simulink model "Open_loop_BPS_comparsion2"  (R2023b)
settings: Solver=VariableStepAuto  StartTime=0.0  StopTime=10.0  RelTol=1e-3
undefined symbols (not defined in the file): X, Y, Z
libraries: nesl_utility x64, sm_lib x24
(part 1 of 2)
settings Model: Creator=msdbg  LastModifiedBy=msdbg

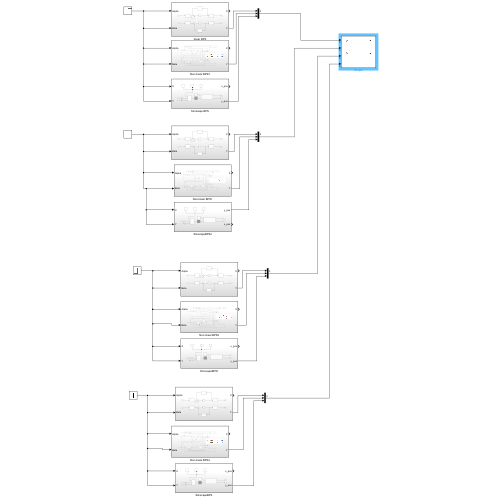
[thumbnail: Simulink's stored preview of the top-level diagram]
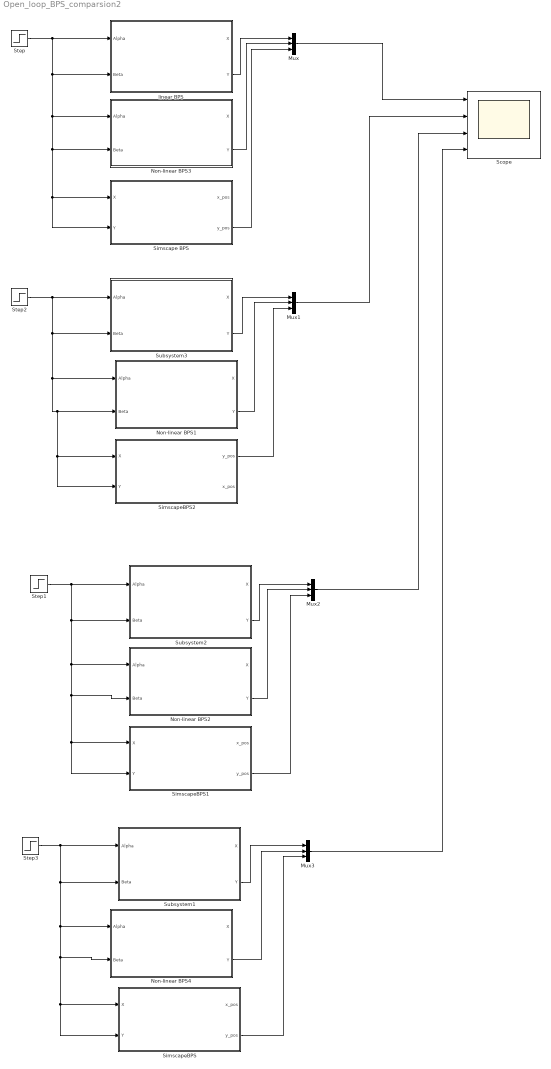
== system Open_loop_BPS_comparsion2 ==
  Mux{,1..3} (4 alike) : Mux  Inputs=3
  Non-linear BPS1 : Subsystem
  Non-linear BPS2 : Subsystem
  Non-linear BPS3 : Subsystem
  Non-linear BPS4 : Subsystem
  Scope : Scope  NumInputPorts=4
  Simscape BPS : Subsystem
  SimscapeBPS : Subsystem
  SimscapeBPS1 : Subsystem
  SimscapeBPS2 : Subsystem
  Step : Step  After=3.14/12  SampleTime=0
  Step1 : Step  After=3.14/8  SampleTime=0
  Step2 : Step  After=3.14/10  SampleTime=0
  Step3 : Step  After=3.14/6  SampleTime=0
  Subsystem1 : Subsystem
  Subsystem2 : Subsystem
  Subsystem3 : Subsystem
  linear BPS : Subsystem
  wires:
  Step3/1 -> Subsystem1/1(Alpha), Subsystem1/2(Beta), Non-linear BPS4/1(Alpha), Non-linear BPS4/2(Beta), SimscapeBPS/2(Y), SimscapeBPS/1(X)
  Mux3/1 -> Scope/4
  Mux/1 -> Scope/1
  Mux1/1 -> Scope/2
  Mux2/1 -> Scope/3
  Step1/1 -> Non-linear BPS2/1(Alpha), Non-linear BPS2/2(Beta), SimscapeBPS1/2(Y), SimscapeBPS1/1(X), Subsystem2/2(Beta), Subsystem2/1(Alpha)
  Step2/1 -> Non-linear BPS1/1(Alpha), Non-linear BPS1/2(Beta), SimscapeBPS2/2(Y), SimscapeBPS2/1(X), Subsystem3/2(Beta), Subsystem3/1(Alpha)
  Step/1 -> Simscape BPS/2(Y), Simscape BPS/1(X), Non-linear BPS3/2(Beta), Non-linear BPS3/1(Alpha), linear BPS/2(Beta), linear BPS/1(Alpha)
  Simscape BPS/2(y_pos) -> Mux/3
  Non-linear BPS1/2(Y) -> Mux1/2
  Non-linear BPS2/2(Y) -> Mux2/2
  Non-linear BPS4/2(Y) -> Mux3/2
  Non-linear BPS3/2(Y) -> Mux/2
  SimscapeBPS2/1(y_pos) -> Mux1/3
  SimscapeBPS1/2(y_pos) -> Mux2/3
  SimscapeBPS/2(y_pos) -> Mux3/3
  Subsystem1/2(Y) -> Mux3/1
  Subsystem2/2(Y) -> Mux2/1
  Subsystem3/2(Y) -> Mux1/1
  linear BPS/2(Y) -> Mux/1

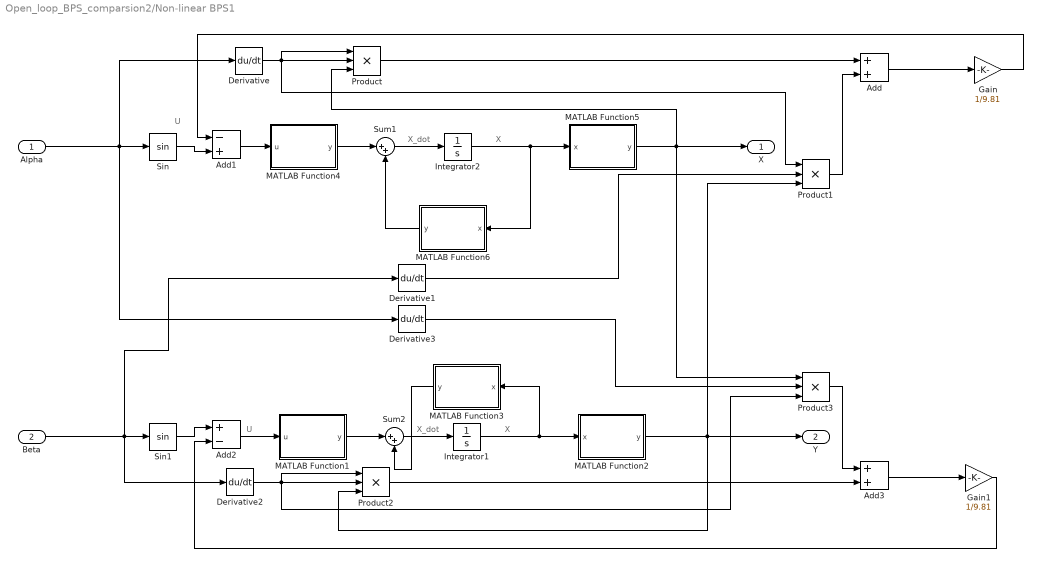
== system Open_loop_BPS_comparsion2/Non-linear BPS1 ==
  note: X
  note: U
  note: X_dot
  note: X_dot
  note: U
  note: X
  Alpha : Inport
  Beta : Inport  Port=2
  Add : Sum
  Add1 : Sum  Inputs=-+
  Add2 : Sum  Inputs=+-
  Add3 : Sum
  Derivative{,1..3} (4 alike) : Derivative
  Gain : Gain  Gain=1/9.81
  Gain1 : Gain  Gain=1/9.81
  Integrator1 : Integrator
  Integrator2 : Integrator
  MATLAB Function1 : MATLAB Function  TreatAsAtomicUnit=on
  MATLAB Function2 : MATLAB Function  TreatAsAtomicUnit=on
  MATLAB Function3 : MATLAB Function  TreatAsAtomicUnit=on
  MATLAB Function4 : MATLAB Function  TreatAsAtomicUnit=on
  MATLAB Function5 : MATLAB Function  TreatAsAtomicUnit=on
  MATLAB Function6 : MATLAB Function  TreatAsAtomicUnit=on
  Product{,1..3} (4 alike) : Product  Inputs=3
  Sin : Trigonometry
  Sin1 : Trigonometry
  Sum1 : Sum  Inputs=|++
  Sum2 : Sum  Inputs=|++
  X : Outport  PortDimensions=1
  Y : Outport  Port=2  PortDimensions=1
  wires:
  Beta/1 -> Sin1/1, Derivative1/1, Derivative2/1
  Alpha/1 -> Derivative3/1, Derivative/1, Sin/1
  Integrator2/1 -> MATLAB Function5/1(x), MATLAB Function6/1(x)
  MATLAB Function6/1(y) -> Sum1/2
  Integrator1/1 -> MATLAB Function2/1(x), MATLAB Function3/1(x)
  Product1/1 -> Add/2
  MATLAB Function3/1(y) -> Sum2/2
  MATLAB Function2/1(y) -> Y/1, Product1/3, Product2/3
  Gain1/1 -> Add2/2
  Derivative1/1 -> Product1/2
  MATLAB Function5/1(y) -> X/1, Product3/1, Product/3
  Add3/1 -> Gain1/1
  MATLAB Function4/1(y) -> Sum1/1
  Sin1/1 -> Add2/1
  Sum1/1 -> Integrator2/1
  MATLAB Function1/1(y) -> Sum2/1
  Derivative2/1 -> Product3/3, Product2/2, Product2/1
  Add/1 -> Gain/1
  Derivative/1 -> Product/1, Product1/1, Product/2
  Add2/1 -> MATLAB Function1/1(u)
  Sin/1 -> Add1/2
  Add1/1 -> MATLAB Function4/1(u)
  Derivative3/1 -> Product3/2
  Product2/1 -> Add3/2
  Sum2/1 -> Integrator1/1
  Product/1 -> Add/1
  Product3/1 -> Add3/1
  Gain/1 -> Add1/1

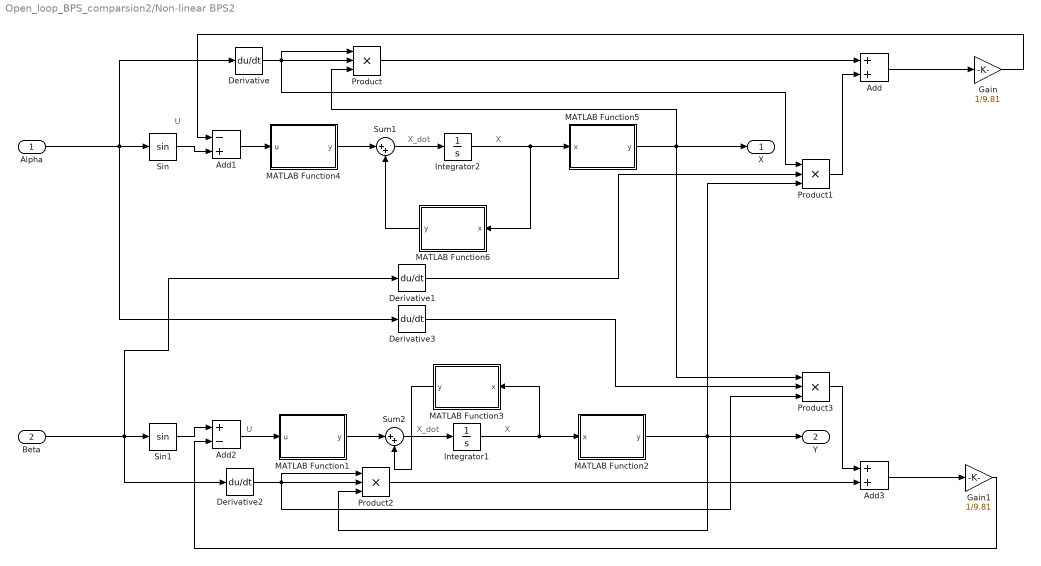
== system Open_loop_BPS_comparsion2/Non-linear BPS2 ==
  note: X
  note: U
  note: X_dot
  note: X_dot
  note: U
  note: X
  Alpha : Inport
  Beta : Inport  Port=2
  Add : Sum
  Add1 : Sum  Inputs=-+
  Add2 : Sum  Inputs=+-
  Add3 : Sum
  Derivative{,1..3} (4 alike) : Derivative
  Gain : Gain  Gain=1/9.81
  Gain1 : Gain  Gain=1/9.81
  Integrator1 : Integrator
  Integrator2 : Integrator
  MATLAB Function1 : MATLAB Function  TreatAsAtomicUnit=on
  MATLAB Function2 : MATLAB Function  TreatAsAtomicUnit=on
  MATLAB Function3 : MATLAB Function  TreatAsAtomicUnit=on
  MATLAB Function4 : MATLAB Function  TreatAsAtomicUnit=on
  MATLAB Function5 : MATLAB Function  TreatAsAtomicUnit=on
  MATLAB Function6 : MATLAB Function  TreatAsAtomicUnit=on
  Product{,1..3} (4 alike) : Product  Inputs=3
  Sin : Trigonometry
  Sin1 : Trigonometry
  Sum1 : Sum  Inputs=|++
  Sum2 : Sum  Inputs=|++
  X : Outport  PortDimensions=1
  Y : Outport  Port=2  PortDimensions=1
  wires:
  Beta/1 -> Sin1/1, Derivative1/1, Derivative2/1
  Alpha/1 -> Derivative3/1, Derivative/1, Sin/1
  Integrator2/1 -> MATLAB Function5/1(x), MATLAB Function6/1(x)
  MATLAB Function6/1(y) -> Sum1/2
  Integrator1/1 -> MATLAB Function2/1(x), MATLAB Function3/1(x)
  Product1/1 -> Add/2
  MATLAB Function3/1(y) -> Sum2/2
  MATLAB Function2/1(y) -> Y/1, Product1/3, Product2/3
  Gain1/1 -> Add2/2
  Derivative1/1 -> Product1/2
  MATLAB Function5/1(y) -> X/1, Product3/1, Product/3
  Add3/1 -> Gain1/1
  MATLAB Function4/1(y) -> Sum1/1
  Sin1/1 -> Add2/1
  Sum1/1 -> Integrator2/1
  MATLAB Function1/1(y) -> Sum2/1
  Derivative2/1 -> Product3/3, Product2/2, Product2/1
  Add/1 -> Gain/1
  Derivative/1 -> Product/1, Product1/1, Product/2
  Add2/1 -> MATLAB Function1/1(u)
  Sin/1 -> Add1/2
  Add1/1 -> MATLAB Function4/1(u)
  Derivative3/1 -> Product3/2
  Product2/1 -> Add3/2
  Sum2/1 -> Integrator1/1
  Product/1 -> Add/1
  Product3/1 -> Add3/1
  Gain/1 -> Add1/1

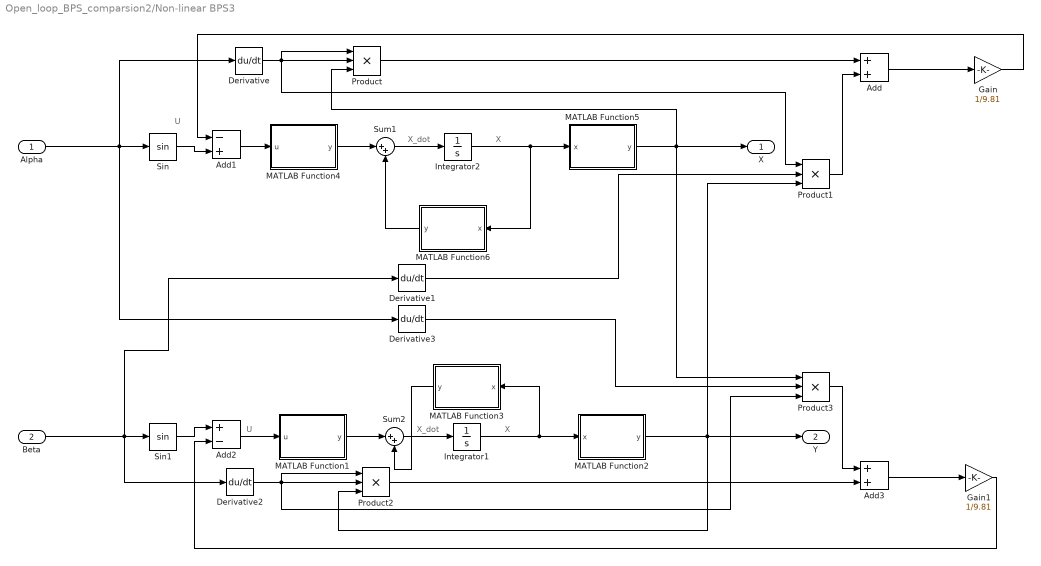
== system Open_loop_BPS_comparsion2/Non-linear BPS3 ==
  note: X
  note: U
  note: X_dot
  note: X_dot
  note: U
  note: X
  Alpha : Inport
  Beta : Inport  Port=2
  Add : Sum
  Add1 : Sum  Inputs=-+
  Add2 : Sum  Inputs=+-
  Add3 : Sum
  Derivative{,1..3} (4 alike) : Derivative
  Gain : Gain  Gain=1/9.81
  Gain1 : Gain  Gain=1/9.81
  Integrator1 : Integrator
  Integrator2 : Integrator
  MATLAB Function1 : MATLAB Function  TreatAsAtomicUnit=on
  MATLAB Function2 : MATLAB Function  TreatAsAtomicUnit=on
  MATLAB Function3 : MATLAB Function  TreatAsAtomicUnit=on
  MATLAB Function4 : MATLAB Function  TreatAsAtomicUnit=on
  MATLAB Function5 : MATLAB Function  TreatAsAtomicUnit=on
  MATLAB Function6 : MATLAB Function  TreatAsAtomicUnit=on
  Product{,1..3} (4 alike) : Product  Inputs=3
  Sin : Trigonometry
  Sin1 : Trigonometry
  Sum1 : Sum  Inputs=|++
  Sum2 : Sum  Inputs=|++
  X : Outport  PortDimensions=1
  Y : Outport  Port=2  PortDimensions=1
  wires:
  Beta/1 -> Sin1/1, Derivative1/1, Derivative2/1
  Alpha/1 -> Derivative3/1, Derivative/1, Sin/1
  Integrator2/1 -> MATLAB Function5/1(x), MATLAB Function6/1(x)
  MATLAB Function6/1(y) -> Sum1/2
  Integrator1/1 -> MATLAB Function2/1(x), MATLAB Function3/1(x)
  Product1/1 -> Add/2
  MATLAB Function3/1(y) -> Sum2/2
  MATLAB Function2/1(y) -> Y/1, Product1/3, Product2/3
  Gain1/1 -> Add2/2
  Derivative1/1 -> Product1/2
  MATLAB Function5/1(y) -> X/1, Product3/1, Product/3
  Add3/1 -> Gain1/1
  MATLAB Function4/1(y) -> Sum1/1
  Sin1/1 -> Add2/1
  Sum1/1 -> Integrator2/1
  MATLAB Function1/1(y) -> Sum2/1
  Derivative2/1 -> Product3/3, Product2/2, Product2/1
  Add/1 -> Gain/1
  Derivative/1 -> Product/1, Product1/1, Product/2
  Add2/1 -> MATLAB Function1/1(u)
  Sin/1 -> Add1/2
  Add1/1 -> MATLAB Function4/1(u)
  Derivative3/1 -> Product3/2
  Product2/1 -> Add3/2
  Sum2/1 -> Integrator1/1
  Product/1 -> Add/1
  Product3/1 -> Add3/1
  Gain/1 -> Add1/1

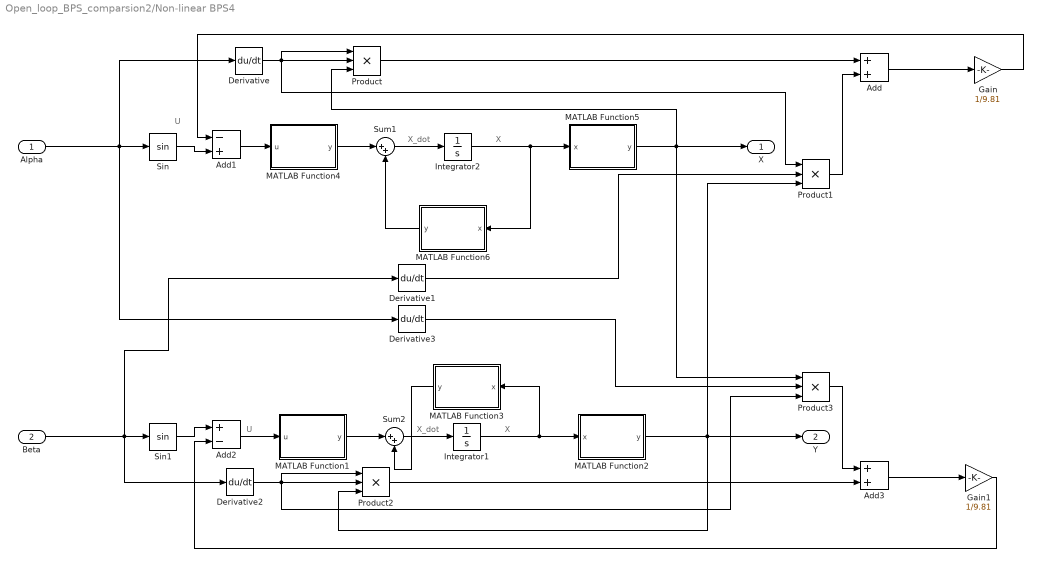
== system Open_loop_BPS_comparsion2/Non-linear BPS4 ==
  note: X
  note: U
  note: X_dot
  note: X_dot
  note: U
  note: X
  Alpha : Inport
  Beta : Inport  Port=2
  Add : Sum
  Add1 : Sum  Inputs=-+
  Add2 : Sum  Inputs=+-
  Add3 : Sum
  Derivative{,1..3} (4 alike) : Derivative
  Gain : Gain  Gain=1/9.81
  Gain1 : Gain  Gain=1/9.81
  Integrator1 : Integrator
  Integrator2 : Integrator
  MATLAB Function1 : MATLAB Function  TreatAsAtomicUnit=on
  MATLAB Function2 : MATLAB Function  TreatAsAtomicUnit=on
  MATLAB Function3 : MATLAB Function  TreatAsAtomicUnit=on
  MATLAB Function4 : MATLAB Function  TreatAsAtomicUnit=on
  MATLAB Function5 : MATLAB Function  TreatAsAtomicUnit=on
  MATLAB Function6 : MATLAB Function  TreatAsAtomicUnit=on
  Product{,1..3} (4 alike) : Product  Inputs=3
  Sin : Trigonometry
  Sin1 : Trigonometry
  Sum1 : Sum  Inputs=|++
  Sum2 : Sum  Inputs=|++
  X : Outport  PortDimensions=1
  Y : Outport  Port=2  PortDimensions=1
  wires:
  Beta/1 -> Sin1/1, Derivative1/1, Derivative2/1
  Alpha/1 -> Derivative3/1, Derivative/1, Sin/1
  Integrator2/1 -> MATLAB Function5/1(x), MATLAB Function6/1(x)
  MATLAB Function6/1(y) -> Sum1/2
  Integrator1/1 -> MATLAB Function2/1(x), MATLAB Function3/1(x)
  Product1/1 -> Add/2
  MATLAB Function3/1(y) -> Sum2/2
  MATLAB Function2/1(y) -> Y/1, Product1/3, Product2/3
  Gain1/1 -> Add2/2
  Derivative1/1 -> Product1/2
  MATLAB Function5/1(y) -> X/1, Product3/1, Product/3
  Add3/1 -> Gain1/1
  MATLAB Function4/1(y) -> Sum1/1
  Sin1/1 -> Add2/1
  Sum1/1 -> Integrator2/1
  MATLAB Function1/1(y) -> Sum2/1
  Derivative2/1 -> Product3/3, Product2/2, Product2/1
  Add/1 -> Gain/1
  Derivative/1 -> Product/1, Product1/1, Product/2
  Add2/1 -> MATLAB Function1/1(u)
  Sin/1 -> Add1/2
  Add1/1 -> MATLAB Function4/1(u)
  Derivative3/1 -> Product3/2
  Product2/1 -> Add3/2
  Sum2/1 -> Integrator1/1
  Product/1 -> Add/1
  Product3/1 -> Add3/1
  Gain/1 -> Add1/1

== system Open_loop_BPS_comparsion2/Simscape BPS ==
  X : Inport
  Y : Inport  Port=2
  Ball : sm_lib/Body Elements/Spherical Solid  GraphicAmbientColor=[0.15 0.15 0.15 1.0]  BasedOnType=Mass  CenterOfMass=[0 0 0]  CenterOfMassUnits=m  GraphicDiffuseColor=[0.5 0.5 0.5]  Density=1000  DensityUnits=kg/m^3  DoExposeReferenceFrame=on  GraphicEmissiveColor=[0.0 0.0 0.0 1.0]  ExportEntireGeometry=off  SerializedExposedGeometries=<exposedGeometries/>  SerializedFrames=<Frames/>  MarkerShape=Sphere  MarkerSize=10  GraphicType=FromGeometry  InertiaType=CalculateFromGeometry  Mass=51  MassUnits=g  MomentsOfInertia=[1 1 1]  MomentsOfInertiaUnits=kg*m^2  GraphicOpacity=1.0  ProductsOfInertia=[0 0 0]  ProductsOfInertiaUnits=kg*m^2  GraphicShininess=75  GraphicSpecularColor=[0.5 0.5 0.5 1.0]  SphereRadius=2.54/2  SphereRadiusUnits=cm  GraphicVisPropType=SimpleVisualProperties
  Ball Plate Interaction : Subsystem
  Mechanism Configuration : sm_lib/Utilities/Mechanism Configuration  UniformGravity=Constant  GravityVector=[0 0 -9.81]  GravityVectorUnits=m/s^2  LinearizationDelta=0.001  JointModeTransitionNonlinearIterations=2
  Plate : Subsystem
  Simulink-PS Converter : nesl_utility/Simulink-PS Converter  PhysicalDomain=network_engine_domain  SubClassName=ps_input  LeftPortType=input  RightPortType=output  PseudoPeriodic=off  Frequencies=[]  NoiseDistribution=none  NoiseParameters=[]  Unit=1  AffineConversion=off  FilteringAndDerivatives=zero  SimscapeFilterOrder=1  InputFilterTimeConstant=0.001  UdotUserProvided=0
  Simulink-PS Converter1 : nesl_utility/Simulink-PS Converter  PhysicalDomain=network_engine_domain  SubClassName=ps_input  LeftPortType=input  RightPortType=output  PseudoPeriodic=off  Frequencies=[]  NoiseDistribution=none  NoiseParameters=[]  Unit=1  AffineConversion=off  FilteringAndDerivatives=zero  SimscapeFilterOrder=1  InputFilterTimeConstant=0.001  UdotUserProvided=0
  Solver Configuration : nesl_utility/Solver Configuration  PhysicalDomain=network_engine_domain  SubClassName=solver  LeftPortType=input  RightPortType=generic  Tones=[]  Harmonics=[]  SimulateNoise=off  Profile=off  UseLocalSampling=off  EnableSwitchedLinearOptims=on  FrequencyDomain=off  UseCCode=off  RelTol=0.001  AbsTol=1e-06  MinStep=1e-09  ToWorkspace=off  RevertToSquareIcSolve=off  NumHomotopyIterations=100  PhasorMode=off  PhasorModeNumHarmonics=1  ConsistencySolver=NEWTON_FTOL  IndexReductionMethod=DerivativeReplacement  DoDC=off  ResidualTolerance=1e-9  ConsistencyTolSource=GLOBAL  ConsistencyAbsTol=0.001  ConsistencyRelTol=0.001  ConsistencyTolFactor=0.001  UseLocalSolver=off  LocalSolverChoice=NE_BACKWARD_EULER_ADVANCER  ResolveIndetEquations=on  FunctionEvalNumThread=1  LocalSolverSampleTime=.001  DoFixedCost=off  MaxNonlinIter=3  MaxModeIter=2  ComputeImpulses=off  ImpulseIterations=2  LinearAlgebra=Sparse  LinearAlgebraNumThread=0  EquationFormulation=NE_TIME_EF  DelaysMemoryBudget=1024  AutomaticFiltering=on  FilteringTimeConstant=0.001  PartitionStorageMethod=AS_NEEDED  PartitionMemoryBudget=1024  PartitionMethod=FAST  MultibodyUseLocalSolver=off  MultibodyLocalSolverChoice=ODE1  MultibodyLocalSolverSampleTime=0.001
  Universal Joint : sm_lib/Joints/Universal Joint  JointMode=Normal  SenseConstraintForce=off  SenseConstraintForceX=off  SenseConstraintForceY=off  SenseConstraintForceZ=off  SenseConstraintTorque=off  SenseConstraintTorqueX=off  SenseConstraintTorqueY=off  SenseConstraintTorqueZ=off  SenseTotalForce=off  SenseTotalForceX=off  SenseTotalForceY=off  SenseTotalForceZ=off  SenseTotalTorque=off  SenseTotalTorqueX=off  SenseTotalTorqueY=off  SenseTotalTorqueZ=off  CompositeWrenchDir=FollowerOnBase  CompositeWrenchFrame=BaseFrame  RxEquilibriumPosition=0  RxEquilibriumPositionUnits=deg  RxSpringStiffness=0  RxSpringStiffnessUnits=N*m/deg  RxDampingCoefficient=0  RxDampingCoefficientUnits=N*m/(deg/s)  RxTorqueActuationMode=ComputedTorque  RxMotionActuationMode=InputMotion  RxSensePosition=off  RxSenseVelocity=off  RxSenseAcceleration=off  RxSenseTorqueForce=off  RxSenseLowerLimitTorqueForce=off  RxSenseUpperLimitTorqueForce=off  RxLowerLimitSpecify=off  RxLowerLimitBound=-90  RxLowerLimitBoundUnits=deg  RxLowerLimitStiffness=1e4  RxLowerLimitStiffnessUnits=N*m/deg  RxLowerLimitDamping=10  RxLowerLimitDampingUnits=N*m/(deg/s)  RxLowerLimitTransitionRegionWidth=0.1  RxLowerLimitTransitionRegionWidthUnits=deg  RxUpperLimitSpecify=off  RxUpperLimitBound=90  RxUpperLimitBoundUnits=deg  RxUpperLimitStiffness=1e4  RxUpperLimitStiffnessUnits=N*m/deg  RxUpperLimitDamping=10  RxUpperLimitDampingUnits=N*m/(deg/s)  RxUpperLimitTransitionRegionWidth=0.1  RxUpperLimitTransitionRegionWidthUnits=deg  RxPositionTargetSpecify=off  RxPositionTargetPriority=High  RxPositionTargetValue=0  RxPositionTargetValueUnits=deg  RxVelocityTargetSpecify=off  RxVelocityTargetPriority=High  RxVelocityTargetValue=0  RxVelocityTargetValueUnits=deg/s  RyEquilibriumPosition=0  RyEquilibriumPositionUnits=deg  RySpringStiffness=0  RySpringStiffnessUnits=N*m/deg  RyDampingCoefficient=0  RyDampingCoefficientUnits=N*m/(deg/s)  RyTorqueActuationMode=ComputedTorque  RyMotionActuationMode=InputMotion  RySensePosition=off  RySenseVelocity=off  RySenseAcceleration=off  RySenseTorqueForce=off  RySenseLowerLimitTorqueForce=off  RySenseUpperLimitTorqueForce=off  RyLowerLimitSpecify=off  RyLowerLimitBound=-90  RyLowerLimitBoundUnits=deg  RyLowerLimitStiffness=1e4  RyLowerLimitStiffnessUnits=N*m/deg  RyLowerLimitDamping=10  RyLowerLimitDampingUnits=N*m/(deg/s)  RyLowerLimitTransitionRegionWidth=0.1  RyLowerLimitTransitionRegionWidthUnits=deg  RyUpperLimitSpecify=off  RyUpperLimitBound=90  RyUpperLimitBoundUnits=deg  RyUpperLimitStiffness=1e4  RyUpperLimitStiffnessUnits=N*m/deg  RyUpperLimitDamping=10  RyUpperLimitDampingUnits=N*m/(deg/s)  RyUpperLimitTransitionRegionWidth=0.1  RyUpperLimitTransitionRegionWidthUnits=deg  RyPositionTargetSpecify=off  RyPositionTargetPriority=High  RyPositionTargetValue=0  RyPositionTargetValueUnits=deg  RyVelocityTargetSpecify=off  RyVelocityTargetPriority=High  RyVelocityTargetValue=0  RyVelocityTargetValueUnits=deg/s
  World Frame : sm_lib/Frames and Transforms/World Frame
  x_pos : Outport  VectorParamsAs1DForOutWhenUnconnected=off
  y_pos : Outport  Port=2  VectorParamsAs1DForOutWhenUnconnected=off
  wires:
  Ball Plate Interaction/2(y_pos) -> y_pos/1
  X/1 -> Simulink-PS Converter/1
  Y/1 -> Simulink-PS Converter1/1
  Ball Plate Interaction/1(x_pos) -> x_pos/1
  connections:
  Plate/RConn1 -- Ball Plate Interaction/LConn2
  Mechanism Configuration/RConn1 -- Solver Configuration/RConn1 -- Universal Joint/LConn1 -- World Frame/RConn1
  Simulink-PS Converter/RConn1 -- Universal Joint/LConn2
  Plate/LConn1 -- Universal Joint/RConn1
  Simulink-PS Converter1/RConn1 -- Universal Joint/LConn3
  Ball Plate Interaction/LConn1 -- Ball/RConn1

== system Open_loop_BPS_comparsion2/SimscapeBPS ==
  X : Inport
  Y : Inport  Port=2
  Ball : sm_lib/Body Elements/Spherical Solid  GraphicAmbientColor=[0.15 0.15 0.15 1.0]  BasedOnType=Mass  CenterOfMass=[0 0 0]  CenterOfMassUnits=m  GraphicDiffuseColor=[0.5 0.5 0.5]  Density=1000  DensityUnits=kg/m^3  DoExposeReferenceFrame=on  GraphicEmissiveColor=[0.0 0.0 0.0 1.0]  ExportEntireGeometry=off  SerializedExposedGeometries=<exposedGeometries/>  SerializedFrames=<Frames/>  MarkerShape=Sphere  MarkerSize=10  GraphicType=FromGeometry  InertiaType=CalculateFromGeometry  Mass=51  MassUnits=g  MomentsOfInertia=[1 1 1]  MomentsOfInertiaUnits=kg*m^2  GraphicOpacity=1.0  ProductsOfInertia=[0 0 0]  ProductsOfInertiaUnits=kg*m^2  GraphicShininess=75  GraphicSpecularColor=[0.5 0.5 0.5 1.0]  SphereRadius=2.54/2  SphereRadiusUnits=cm  GraphicVisPropType=SimpleVisualProperties
  Ball Plate Interaction : Subsystem
  Mechanism Configuration : sm_lib/Utilities/Mechanism Configuration  UniformGravity=Constant  GravityVector=[0 0 -9.81]  GravityVectorUnits=m/s^2  LinearizationDelta=0.001  JointModeTransitionNonlinearIterations=2
  Plate : Subsystem
  Simulink-PS Converter : nesl_utility/Simulink-PS Converter  PhysicalDomain=network_engine_domain  SubClassName=ps_input  LeftPortType=input  RightPortType=output  PseudoPeriodic=off  Frequencies=[]  NoiseDistribution=none  NoiseParameters=[]  Unit=1  AffineConversion=off  FilteringAndDerivatives=zero  SimscapeFilterOrder=1  InputFilterTimeConstant=0.001  UdotUserProvided=0
  Simulink-PS Converter1 : nesl_utility/Simulink-PS Converter  PhysicalDomain=network_engine_domain  SubClassName=ps_input  LeftPortType=input  RightPortType=output  PseudoPeriodic=off  Frequencies=[]  NoiseDistribution=none  NoiseParameters=[]  Unit=1  AffineConversion=off  FilteringAndDerivatives=zero  SimscapeFilterOrder=1  InputFilterTimeConstant=0.001  UdotUserProvided=0
  Solver Configuration : nesl_utility/Solver Configuration  PhysicalDomain=network_engine_domain  SubClassName=solver  LeftPortType=input  RightPortType=generic  Tones=[]  Harmonics=[]  SimulateNoise=off  Profile=off  UseLocalSampling=off  EnableSwitchedLinearOptims=on  FrequencyDomain=off  UseCCode=off  RelTol=0.001  AbsTol=1e-06  MinStep=1e-09  ToWorkspace=off  RevertToSquareIcSolve=off  NumHomotopyIterations=100  PhasorMode=off  PhasorModeNumHarmonics=1  ConsistencySolver=NEWTON_FTOL  IndexReductionMethod=DerivativeReplacement  DoDC=off  ResidualTolerance=1e-9  ConsistencyTolSource=GLOBAL  ConsistencyAbsTol=0.001  ConsistencyRelTol=0.001  ConsistencyTolFactor=0.001  UseLocalSolver=off  LocalSolverChoice=NE_BACKWARD_EULER_ADVANCER  ResolveIndetEquations=on  FunctionEvalNumThread=1  LocalSolverSampleTime=.001  DoFixedCost=off  MaxNonlinIter=3  MaxModeIter=2  ComputeImpulses=off  ImpulseIterations=2  LinearAlgebra=Sparse  LinearAlgebraNumThread=0  EquationFormulation=NE_TIME_EF  DelaysMemoryBudget=1024  AutomaticFiltering=on  FilteringTimeConstant=0.001  PartitionStorageMethod=AS_NEEDED  PartitionMemoryBudget=1024  PartitionMethod=FAST  MultibodyUseLocalSolver=off  MultibodyLocalSolverChoice=ODE1  MultibodyLocalSolverSampleTime=0.001
  Universal Joint : sm_lib/Joints/Universal Joint  JointMode=Normal  SenseConstraintForce=off  SenseConstraintForceX=off  SenseConstraintForceY=off  SenseConstraintForceZ=off  SenseConstraintTorque=off  SenseConstraintTorqueX=off  SenseConstraintTorqueY=off  SenseConstraintTorqueZ=off  SenseTotalForce=off  SenseTotalForceX=off  SenseTotalForceY=off  SenseTotalForceZ=off  SenseTotalTorque=off  SenseTotalTorqueX=off  SenseTotalTorqueY=off  SenseTotalTorqueZ=off  CompositeWrenchDir=FollowerOnBase  CompositeWrenchFrame=BaseFrame  RxEquilibriumPosition=0  RxEquilibriumPositionUnits=deg  RxSpringStiffness=0  RxSpringStiffnessUnits=N*m/deg  RxDampingCoefficient=0  RxDampingCoefficientUnits=N*m/(deg/s)  RxTorqueActuationMode=ComputedTorque  RxMotionActuationMode=InputMotion  RxSensePosition=off  RxSenseVelocity=off  RxSenseAcceleration=off  RxSenseTorqueForce=off  RxSenseLowerLimitTorqueForce=off  RxSenseUpperLimitTorqueForce=off  RxLowerLimitSpecify=off  RxLowerLimitBound=-90  RxLowerLimitBoundUnits=deg  RxLowerLimitStiffness=1e4  RxLowerLimitStiffnessUnits=N*m/deg  RxLowerLimitDamping=10  RxLowerLimitDampingUnits=N*m/(deg/s)  RxLowerLimitTransitionRegionWidth=0.1  RxLowerLimitTransitionRegionWidthUnits=deg  RxUpperLimitSpecify=off  RxUpperLimitBound=90  RxUpperLimitBoundUnits=deg  RxUpperLimitStiffness=1e4  RxUpperLimitStiffnessUnits=N*m/deg  RxUpperLimitDamping=10  RxUpperLimitDampingUnits=N*m/(deg/s)  RxUpperLimitTransitionRegionWidth=0.1  RxUpperLimitTransitionRegionWidthUnits=deg  RxPositionTargetSpecify=off  RxPositionTargetPriority=High  RxPositionTargetValue=0  RxPositionTargetValueUnits=deg  RxVelocityTargetSpecify=off  RxVelocityTargetPriority=High  RxVelocityTargetValue=0  RxVelocityTargetValueUnits=deg/s  RyEquilibriumPosition=0  RyEquilibriumPositionUnits=deg  RySpringStiffness=0  RySpringStiffnessUnits=N*m/deg  RyDampingCoefficient=0  RyDampingCoefficientUnits=N*m/(deg/s)  RyTorqueActuationMode=ComputedTorque  RyMotionActuationMode=InputMotion  RySensePosition=off  RySenseVelocity=off  RySenseAcceleration=off  RySenseTorqueForce=off  RySenseLowerLimitTorqueForce=off  RySenseUpperLimitTorqueForce=off  RyLowerLimitSpecify=off  RyLowerLimitBound=-90  RyLowerLimitBoundUnits=deg  RyLowerLimitStiffness=1e4  RyLowerLimitStiffnessUnits=N*m/deg  RyLowerLimitDamping=10  RyLowerLimitDampingUnits=N*m/(deg/s)  RyLowerLimitTransitionRegionWidth=0.1  RyLowerLimitTransitionRegionWidthUnits=deg  RyUpperLimitSpecify=off  RyUpperLimitBound=90  RyUpperLimitBoundUnits=deg  RyUpperLimitStiffness=1e4  RyUpperLimitStiffnessUnits=N*m/deg  RyUpperLimitDamping=10  RyUpperLimitDampingUnits=N*m/(deg/s)  RyUpperLimitTransitionRegionWidth=0.1  RyUpperLimitTransitionRegionWidthUnits=deg  RyPositionTargetSpecify=off  RyPositionTargetPriority=High  RyPositionTargetValue=0  RyPositionTargetValueUnits=deg  RyVelocityTargetSpecify=off  RyVelocityTargetPriority=High  RyVelocityTargetValue=0  RyVelocityTargetValueUnits=deg/s
  World Frame : sm_lib/Frames and Transforms/World Frame
  x_pos : Outport  VectorParamsAs1DForOutWhenUnconnected=off
  y_pos : Outport  Port=2  VectorParamsAs1DForOutWhenUnconnected=off
  wires:
  Ball Plate Interaction/2(y_pos) -> y_pos/1
  X/1 -> Simulink-PS Converter/1
  Y/1 -> Simulink-PS Converter1/1
  Ball Plate Interaction/1(x_pos) -> x_pos/1
  connections:
  Plate/RConn1 -- Ball Plate Interaction/LConn2
  Mechanism Configuration/RConn1 -- Solver Configuration/RConn1 -- Universal Joint/LConn1 -- World Frame/RConn1
  Simulink-PS Converter/RConn1 -- Universal Joint/LConn2
  Plate/LConn1 -- Universal Joint/RConn1
  Simulink-PS Converter1/RConn1 -- Universal Joint/LConn3
  Ball Plate Interaction/LConn1 -- Ball/RConn1

== system Open_loop_BPS_comparsion2/SimscapeBPS1 ==
  X : Inport
  Y : Inport  Port=2
  Ball : sm_lib/Body Elements/Spherical Solid  GraphicAmbientColor=[0.15 0.15 0.15 1.0]  BasedOnType=Mass  CenterOfMass=[0 0 0]  CenterOfMassUnits=m  GraphicDiffuseColor=[0.5 0.5 0.5]  Density=1000  DensityUnits=kg/m^3  DoExposeReferenceFrame=on  GraphicEmissiveColor=[0.0 0.0 0.0 1.0]  ExportEntireGeometry=off  SerializedExposedGeometries=<exposedGeometries/>  SerializedFrames=<Frames/>  MarkerShape=Sphere  MarkerSize=10  GraphicType=FromGeometry  InertiaType=CalculateFromGeometry  Mass=51  MassUnits=g  MomentsOfInertia=[1 1 1]  MomentsOfInertiaUnits=kg*m^2  GraphicOpacity=1.0  ProductsOfInertia=[0 0 0]  ProductsOfInertiaUnits=kg*m^2  GraphicShininess=75  GraphicSpecularColor=[0.5 0.5 0.5 1.0]  SphereRadius=2.54/2  SphereRadiusUnits=cm  GraphicVisPropType=SimpleVisualProperties
  Ball Plate Interaction : Subsystem
  Mechanism Configuration : sm_lib/Utilities/Mechanism Configuration  UniformGravity=Constant  GravityVector=[0 0 -9.81]  GravityVectorUnits=m/s^2  LinearizationDelta=0.001  JointModeTransitionNonlinearIterations=2
  Plate : Subsystem
  Simulink-PS Converter : nesl_utility/Simulink-PS Converter  PhysicalDomain=network_engine_domain  SubClassName=ps_input  LeftPortType=input  RightPortType=output  PseudoPeriodic=off  Frequencies=[]  NoiseDistribution=none  NoiseParameters=[]  Unit=1  AffineConversion=off  FilteringAndDerivatives=zero  SimscapeFilterOrder=1  InputFilterTimeConstant=0.001  UdotUserProvided=0
  Simulink-PS Converter1 : nesl_utility/Simulink-PS Converter  PhysicalDomain=network_engine_domain  SubClassName=ps_input  LeftPortType=input  RightPortType=output  PseudoPeriodic=off  Frequencies=[]  NoiseDistribution=none  NoiseParameters=[]  Unit=1  AffineConversion=off  FilteringAndDerivatives=zero  SimscapeFilterOrder=1  InputFilterTimeConstant=0.001  UdotUserProvided=0
  Solver Configuration : nesl_utility/Solver Configuration  PhysicalDomain=network_engine_domain  SubClassName=solver  LeftPortType=input  RightPortType=generic  Tones=[]  Harmonics=[]  SimulateNoise=off  Profile=off  UseLocalSampling=off  EnableSwitchedLinearOptims=on  FrequencyDomain=off  UseCCode=off  RelTol=0.001  AbsTol=1e-06  MinStep=1e-09  ToWorkspace=off  RevertToSquareIcSolve=off  NumHomotopyIterations=100  PhasorMode=off  PhasorModeNumHarmonics=1  ConsistencySolver=NEWTON_FTOL  IndexReductionMethod=DerivativeReplacement  DoDC=off  ResidualTolerance=1e-9  ConsistencyTolSource=GLOBAL  ConsistencyAbsTol=0.001  ConsistencyRelTol=0.001  ConsistencyTolFactor=0.001  UseLocalSolver=off  LocalSolverChoice=NE_BACKWARD_EULER_ADVANCER  ResolveIndetEquations=on  FunctionEvalNumThread=1  LocalSolverSampleTime=.001  DoFixedCost=off  MaxNonlinIter=3  MaxModeIter=2  ComputeImpulses=off  ImpulseIterations=2  LinearAlgebra=Sparse  LinearAlgebraNumThread=0  EquationFormulation=NE_TIME_EF  DelaysMemoryBudget=1024  AutomaticFiltering=on  FilteringTimeConstant=0.001  PartitionStorageMethod=AS_NEEDED  PartitionMemoryBudget=1024  PartitionMethod=FAST  MultibodyUseLocalSolver=off  MultibodyLocalSolverChoice=ODE1  MultibodyLocalSolverSampleTime=0.001
  Universal Joint : sm_lib/Joints/Universal Joint  JointMode=Normal  SenseConstraintForce=off  SenseConstraintForceX=off  SenseConstraintForceY=off  SenseConstraintForceZ=off  SenseConstraintTorque=off  SenseConstraintTorqueX=off  SenseConstraintTorqueY=off  SenseConstraintTorqueZ=off  SenseTotalForce=off  SenseTotalForceX=off  SenseTotalForceY=off  SenseTotalForceZ=off  SenseTotalTorque=off  SenseTotalTorqueX=off  SenseTotalTorqueY=off  SenseTotalTorqueZ=off  CompositeWrenchDir=FollowerOnBase  CompositeWrenchFrame=BaseFrame  RxEquilibriumPosition=0  RxEquilibriumPositionUnits=deg  RxSpringStiffness=0  RxSpringStiffnessUnits=N*m/deg  RxDampingCoefficient=0  RxDampingCoefficientUnits=N*m/(deg/s)  RxTorqueActuationMode=ComputedTorque  RxMotionActuationMode=InputMotion  RxSensePosition=off  RxSenseVelocity=off  RxSenseAcceleration=off  RxSenseTorqueForce=off  RxSenseLowerLimitTorqueForce=off  RxSenseUpperLimitTorqueForce=off  RxLowerLimitSpecify=off  RxLowerLimitBound=-90  RxLowerLimitBoundUnits=deg  RxLowerLimitStiffness=1e4  RxLowerLimitStiffnessUnits=N*m/deg  RxLowerLimitDamping=10  RxLowerLimitDampingUnits=N*m/(deg/s)  RxLowerLimitTransitionRegionWidth=0.1  RxLowerLimitTransitionRegionWidthUnits=deg  RxUpperLimitSpecify=off  RxUpperLimitBound=90  RxUpperLimitBoundUnits=deg  RxUpperLimitStiffness=1e4  RxUpperLimitStiffnessUnits=N*m/deg  RxUpperLimitDamping=10  RxUpperLimitDampingUnits=N*m/(deg/s)  RxUpperLimitTransitionRegionWidth=0.1  RxUpperLimitTransitionRegionWidthUnits=deg  RxPositionTargetSpecify=off  RxPositionTargetPriority=High  RxPositionTargetValue=0  RxPositionTargetValueUnits=deg  RxVelocityTargetSpecify=off  RxVelocityTargetPriority=High  RxVelocityTargetValue=0  RxVelocityTargetValueUnits=deg/s  RyEquilibriumPosition=0  RyEquilibriumPositionUnits=deg  RySpringStiffness=0  RySpringStiffnessUnits=N*m/deg  RyDampingCoefficient=0  RyDampingCoefficientUnits=N*m/(deg/s)  RyTorqueActuationMode=ComputedTorque  RyMotionActuationMode=InputMotion  RySensePosition=off  RySenseVelocity=off  RySenseAcceleration=off  RySenseTorqueForce=off  RySenseLowerLimitTorqueForce=off  RySenseUpperLimitTorqueForce=off  RyLowerLimitSpecify=off  RyLowerLimitBound=-90  RyLowerLimitBoundUnits=deg  RyLowerLimitStiffness=1e4  RyLowerLimitStiffnessUnits=N*m/deg  RyLowerLimitDamping=10  RyLowerLimitDampingUnits=N*m/(deg/s)  RyLowerLimitTransitionRegionWidth=0.1  RyLowerLimitTransitionRegionWidthUnits=deg  RyUpperLimitSpecify=off  RyUpperLimitBound=90  RyUpperLimitBoundUnits=deg  RyUpperLimitStiffness=1e4  RyUpperLimitStiffnessUnits=N*m/deg  RyUpperLimitDamping=10  RyUpperLimitDampingUnits=N*m/(deg/s)  RyUpperLimitTransitionRegionWidth=0.1  RyUpperLimitTransitionRegionWidthUnits=deg  RyPositionTargetSpecify=off  RyPositionTargetPriority=High  RyPositionTargetValue=0  RyPositionTargetValueUnits=deg  RyVelocityTargetSpecify=off  RyVelocityTargetPriority=High  RyVelocityTargetValue=0  RyVelocityTargetValueUnits=deg/s
  World Frame : sm_lib/Frames and Transforms/World Frame
  x_pos : Outport  VectorParamsAs1DForOutWhenUnconnected=off
  y_pos : Outport  Port=2  VectorParamsAs1DForOutWhenUnconnected=off
  wires:
  Ball Plate Interaction/2(y_pos) -> y_pos/1
  X/1 -> Simulink-PS Converter/1
  Y/1 -> Simulink-PS Converter1/1
  Ball Plate Interaction/1(x_pos) -> x_pos/1
  connections:
  Plate/RConn1 -- Ball Plate Interaction/LConn2
  Mechanism Configuration/RConn1 -- Solver Configuration/RConn1 -- Universal Joint/LConn1 -- World Frame/RConn1
  Simulink-PS Converter/RConn1 -- Universal Joint/LConn2
  Plate/LConn1 -- Universal Joint/RConn1
  Simulink-PS Converter1/RConn1 -- Universal Joint/LConn3
  Ball Plate Interaction/LConn1 -- Ball/RConn1

== system Open_loop_BPS_comparsion2/SimscapeBPS2 ==
  X : Inport
  Y : Inport  Port=2
  Ball : sm_lib/Body Elements/Spherical Solid  GraphicAmbientColor=[0.15 0.15 0.15 1.0]  BasedOnType=Mass  CenterOfMass=[0 0 0]  CenterOfMassUnits=m  GraphicDiffuseColor=[0.5 0.5 0.5]  Density=1000  DensityUnits=kg/m^3  DoExposeReferenceFrame=on  GraphicEmissiveColor=[0.0 0.0 0.0 1.0]  ExportEntireGeometry=off  SerializedExposedGeometries=<exposedGeometries/>  SerializedFrames=<Frames/>  MarkerShape=Sphere  MarkerSize=10  GraphicType=FromGeometry  InertiaType=CalculateFromGeometry  Mass=51  MassUnits=g  MomentsOfInertia=[1 1 1]  MomentsOfInertiaUnits=kg*m^2  GraphicOpacity=1.0  ProductsOfInertia=[0 0 0]  ProductsOfInertiaUnits=kg*m^2  GraphicShininess=75  GraphicSpecularColor=[0.5 0.5 0.5 1.0]  SphereRadius=2.54/2  SphereRadiusUnits=cm  GraphicVisPropType=SimpleVisualProperties
  Ball Plate Interaction : Subsystem
  Mechanism Configuration : sm_lib/Utilities/Mechanism Configuration  UniformGravity=Constant  GravityVector=[0 0 -9.81]  GravityVectorUnits=m/s^2  LinearizationDelta=0.001  JointModeTransitionNonlinearIterations=2
  Plate : Subsystem
  Simulink-PS Converter : nesl_utility/Simulink-PS Converter  PhysicalDomain=network_engine_domain  SubClassName=ps_input  LeftPortType=input  RightPortType=output  PseudoPeriodic=off  Frequencies=[]  NoiseDistribution=none  NoiseParameters=[]  Unit=1  AffineConversion=off  FilteringAndDerivatives=zero  SimscapeFilterOrder=1  InputFilterTimeConstant=0.001  UdotUserProvided=0
  Simulink-PS Converter1 : nesl_utility/Simulink-PS Converter  PhysicalDomain=network_engine_domain  SubClassName=ps_input  LeftPortType=input  RightPortType=output  PseudoPeriodic=off  Frequencies=[]  NoiseDistribution=none  NoiseParameters=[]  Unit=1  AffineConversion=off  FilteringAndDerivatives=zero  SimscapeFilterOrder=1  InputFilterTimeConstant=0.001  UdotUserProvided=0
  Solver Configuration : nesl_utility/Solver Configuration  PhysicalDomain=network_engine_domain  SubClassName=solver  LeftPortType=input  RightPortType=generic  Tones=[]  Harmonics=[]  SimulateNoise=off  Profile=off  UseLocalSampling=off  EnableSwitchedLinearOptims=on  FrequencyDomain=off  UseCCode=off  RelTol=0.001  AbsTol=1e-06  MinStep=1e-09  ToWorkspace=off  RevertToSquareIcSolve=off  NumHomotopyIterations=100  PhasorMode=off  PhasorModeNumHarmonics=1  ConsistencySolver=NEWTON_FTOL  IndexReductionMethod=DerivativeReplacement  DoDC=off  ResidualTolerance=1e-9  ConsistencyTolSource=GLOBAL  ConsistencyAbsTol=0.001  ConsistencyRelTol=0.001  ConsistencyTolFactor=0.001  UseLocalSolver=off  LocalSolverChoice=NE_BACKWARD_EULER_ADVANCER  ResolveIndetEquations=on  FunctionEvalNumThread=1  LocalSolverSampleTime=.001  DoFixedCost=off  MaxNonlinIter=3  MaxModeIter=2  ComputeImpulses=off  ImpulseIterations=2  LinearAlgebra=Sparse  LinearAlgebraNumThread=0  EquationFormulation=NE_TIME_EF  DelaysMemoryBudget=1024  AutomaticFiltering=on  FilteringTimeConstant=0.001  PartitionStorageMethod=AS_NEEDED  PartitionMemoryBudget=1024  PartitionMethod=FAST  MultibodyUseLocalSolver=off  MultibodyLocalSolverChoice=ODE1  MultibodyLocalSolverSampleTime=0.001
  Universal Joint : sm_lib/Joints/Universal Joint  JointMode=Normal  SenseConstraintForce=off  SenseConstraintForceX=off  SenseConstraintForceY=off  SenseConstraintForceZ=off  SenseConstraintTorque=off  SenseConstraintTorqueX=off  SenseConstraintTorqueY=off  SenseConstraintTorqueZ=off  SenseTotalForce=off  SenseTotalForceX=off  SenseTotalForceY=off  SenseTotalForceZ=off  SenseTotalTorque=off  SenseTotalTorqueX=off  SenseTotalTorqueY=off  SenseTotalTorqueZ=off  CompositeWrenchDir=FollowerOnBase  CompositeWrenchFrame=BaseFrame  RxEquilibriumPosition=0  RxEquilibriumPositionUnits=deg  RxSpringStiffness=0  RxSpringStiffnessUnits=N*m/deg  RxDampingCoefficient=0  RxDampingCoefficientUnits=N*m/(deg/s)  RxTorqueActuationMode=ComputedTorque  RxMotionActuationMode=InputMotion  RxSensePosition=off  RxSenseVelocity=off  RxSenseAcceleration=off  RxSenseTorqueForce=off  RxSenseLowerLimitTorqueForce=off  RxSenseUpperLimitTorqueForce=off  RxLowerLimitSpecify=off  RxLowerLimitBound=-90  RxLowerLimitBoundUnits=deg  RxLowerLimitStiffness=1e4  RxLowerLimitStiffnessUnits=N*m/deg  RxLowerLimitDamping=10  RxLowerLimitDampingUnits=N*m/(deg/s)  RxLowerLimitTransitionRegionWidth=0.1  RxLowerLimitTransitionRegionWidthUnits=deg  RxUpperLimitSpecify=off  RxUpperLimitBound=90  RxUpperLimitBoundUnits=deg  RxUpperLimitStiffness=1e4  RxUpperLimitStiffnessUnits=N*m/deg  RxUpperLimitDamping=10  RxUpperLimitDampingUnits=N*m/(deg/s)  RxUpperLimitTransitionRegionWidth=0.1  RxUpperLimitTransitionRegionWidthUnits=deg  RxPositionTargetSpecify=off  RxPositionTargetPriority=High  RxPositionTargetValue=0  RxPositionTargetValueUnits=deg  RxVelocityTargetSpecify=off  RxVelocityTargetPriority=High  RxVelocityTargetValue=0  RxVelocityTargetValueUnits=deg/s  RyEquilibriumPosition=0  RyEquilibriumPositionUnits=deg  RySpringStiffness=0  RySpringStiffnessUnits=N*m/deg  RyDampingCoefficient=0  RyDampingCoefficientUnits=N*m/(deg/s)  RyTorqueActuationMode=ComputedTorque  RyMotionActuationMode=InputMotion  RySensePosition=off  RySenseVelocity=off  RySenseAcceleration=off  RySenseTorqueForce=off  RySenseLowerLimitTorqueForce=off  RySenseUpperLimitTorqueForce=off  RyLowerLimitSpecify=off  RyLowerLimitBound=-90  RyLowerLimitBoundUnits=deg  RyLowerLimitStiffness=1e4  RyLowerLimitStiffnessUnits=N*m/deg  RyLowerLimitDamping=10  RyLowerLimitDampingUnits=N*m/(deg/s)  RyLowerLimitTransitionRegionWidth=0.1  RyLowerLimitTransitionRegionWidthUnits=deg  RyUpperLimitSpecify=off  RyUpperLimitBound=90  RyUpperLimitBoundUnits=deg  RyUpperLimitStiffness=1e4  RyUpperLimitStiffnessUnits=N*m/deg  RyUpperLimitDamping=10  RyUpperLimitDampingUnits=N*m/(deg/s)  RyUpperLimitTransitionRegionWidth=0.1  RyUpperLimitTransitionRegionWidthUnits=deg  RyPositionTargetSpecify=off  RyPositionTargetPriority=High  RyPositionTargetValue=0  RyPositionTargetValueUnits=deg  RyVelocityTargetSpecify=off  RyVelocityTargetPriority=High  RyVelocityTargetValue=0  RyVelocityTargetValueUnits=deg/s
  World Frame : sm_lib/Frames and Transforms/World Frame
  y_pos : Outport  VectorParamsAs1DForOutWhenUnconnected=off
  x_pos : Outport  Port=2  VectorParamsAs1DForOutWhenUnconnected=off
  wires:
  Ball Plate Interaction/2(y_pos) -> y_pos/1
  X/1 -> Simulink-PS Converter/1
  Y/1 -> Simulink-PS Converter1/1
  Ball Plate Interaction/1(x_pos) -> x_pos/1
  connections:
  Plate/RConn1 -- Ball Plate Interaction/LConn2
  Mechanism Configuration/RConn1 -- Solver Configuration/RConn1 -- Universal Joint/LConn1 -- World Frame/RConn1
  Simulink-PS Converter/RConn1 -- Universal Joint/LConn2
  Plate/LConn1 -- Universal Joint/RConn1
  Simulink-PS Converter1/RConn1 -- Universal Joint/LConn3
  Ball Plate Interaction/LConn1 -- Ball/RConn1

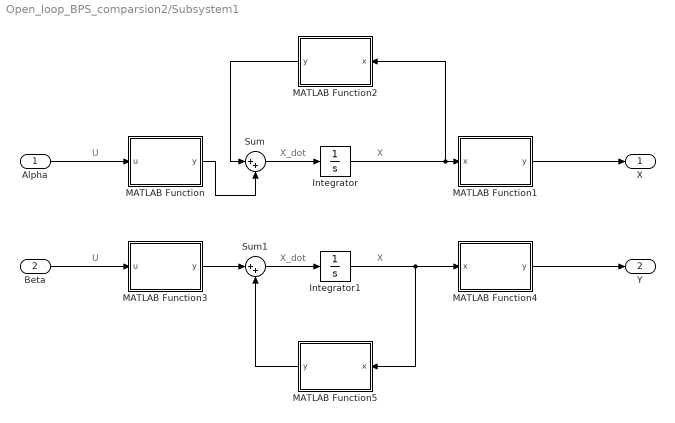
== system Open_loop_BPS_comparsion2/Subsystem1 ==
  note: X_dot
  note: X
  note: U
  note: U
  note: X_dot
  note: X
  Alpha : Inport
  Beta : Inport  Port=2
  Integrator : Integrator
  Integrator1 : Integrator
  MATLAB Function : MATLAB Function  TreatAsAtomicUnit=on
  MATLAB Function1 : MATLAB Function  TreatAsAtomicUnit=on
  MATLAB Function2 : MATLAB Function  TreatAsAtomicUnit=on
  MATLAB Function3 : MATLAB Function  TreatAsAtomicUnit=on
  MATLAB Function4 : MATLAB Function  TreatAsAtomicUnit=on
  MATLAB Function5 : MATLAB Function  TreatAsAtomicUnit=on
  Sum : Sum  Inputs=|++
  Sum1 : Sum  Inputs=|++
  X : Outport
  Y : Outport  Port=2
  wires:
  MATLAB Function2/1(y) -> Sum/1
  MATLAB Function/1(y) -> Sum/2
  MATLAB Function1/1(y) -> X/1
  Sum1/1 -> Integrator1/1
  Integrator/1 -> MATLAB Function2/1(x), MATLAB Function1/1(x)
  Sum/1 -> Integrator/1
  MATLAB Function5/1(y) -> Sum1/2
  MATLAB Function4/1(y) -> Y/1
  Beta/1 -> MATLAB Function3/1(u)
  Integrator1/1 -> MATLAB Function5/1(x), MATLAB Function4/1(x)
  MATLAB Function3/1(y) -> Sum1/1
  Alpha/1 -> MATLAB Function/1(u)

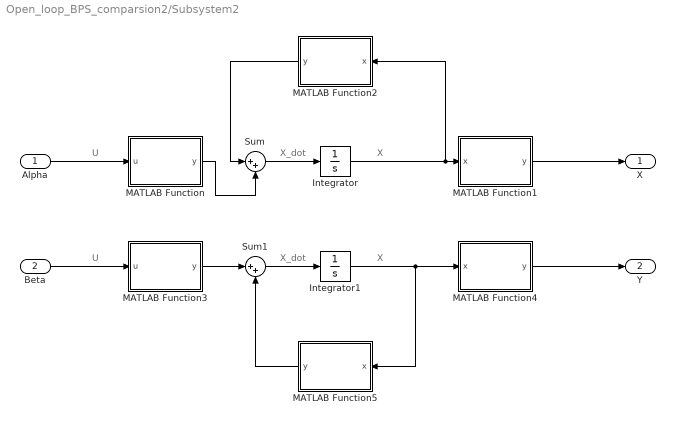
== system Open_loop_BPS_comparsion2/Subsystem2 ==
  note: X_dot
  note: X
  note: U
  note: U
  note: X_dot
  note: X
  Alpha : Inport
  Beta : Inport  Port=2
  Integrator : Integrator
  Integrator1 : Integrator
  MATLAB Function : MATLAB Function  TreatAsAtomicUnit=on
  MATLAB Function1 : MATLAB Function  TreatAsAtomicUnit=on
  MATLAB Function2 : MATLAB Function  TreatAsAtomicUnit=on
  MATLAB Function3 : MATLAB Function  TreatAsAtomicUnit=on
  MATLAB Function4 : MATLAB Function  TreatAsAtomicUnit=on
  MATLAB Function5 : MATLAB Function  TreatAsAtomicUnit=on
  Sum : Sum  Inputs=|++
  Sum1 : Sum  Inputs=|++
  X : Outport
  Y : Outport  Port=2
  wires:
  MATLAB Function2/1(y) -> Sum/1
  MATLAB Function/1(y) -> Sum/2
  MATLAB Function1/1(y) -> X/1
  Sum1/1 -> Integrator1/1
  Integrator/1 -> MATLAB Function2/1(x), MATLAB Function1/1(x)
  Sum/1 -> Integrator/1
  MATLAB Function5/1(y) -> Sum1/2
  MATLAB Function4/1(y) -> Y/1
  Beta/1 -> MATLAB Function3/1(u)
  Integrator1/1 -> MATLAB Function5/1(x), MATLAB Function4/1(x)
  MATLAB Function3/1(y) -> Sum1/1
  Alpha/1 -> MATLAB Function/1(u)

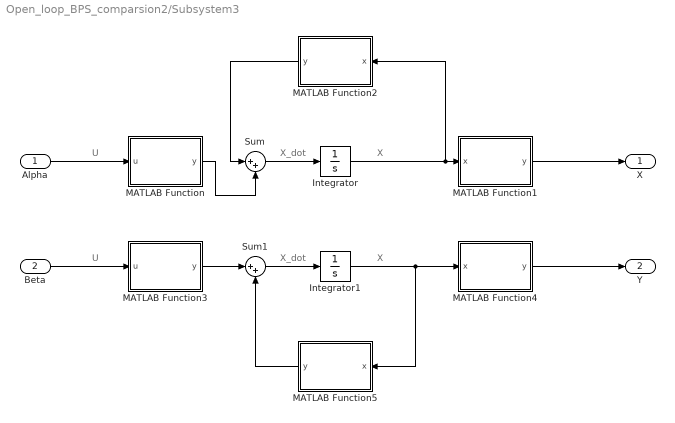
== system Open_loop_BPS_comparsion2/Subsystem3 ==
  note: X_dot
  note: X
  note: U
  note: U
  note: X_dot
  note: X
  Alpha : Inport
  Beta : Inport  Port=2
  Integrator : Integrator
  Integrator1 : Integrator
  MATLAB Function : MATLAB Function  TreatAsAtomicUnit=on
  MATLAB Function1 : MATLAB Function  TreatAsAtomicUnit=on
  MATLAB Function2 : MATLAB Function  TreatAsAtomicUnit=on
  MATLAB Function3 : MATLAB Function  TreatAsAtomicUnit=on
  MATLAB Function4 : MATLAB Function  TreatAsAtomicUnit=on
  MATLAB Function5 : MATLAB Function  TreatAsAtomicUnit=on
  Sum : Sum  Inputs=|++
  Sum1 : Sum  Inputs=|++
  X : Outport
  Y : Outport  Port=2
  wires:
  MATLAB Function2/1(y) -> Sum/1
  MATLAB Function/1(y) -> Sum/2
  MATLAB Function1/1(y) -> X/1
  Sum1/1 -> Integrator1/1
  Integrator/1 -> MATLAB Function2/1(x), MATLAB Function1/1(x)
  Sum/1 -> Integrator/1
  MATLAB Function5/1(y) -> Sum1/2
  MATLAB Function4/1(y) -> Y/1
  Beta/1 -> MATLAB Function3/1(u)
  Integrator1/1 -> MATLAB Function5/1(x), MATLAB Function4/1(x)
  MATLAB Function3/1(y) -> Sum1/1
  Alpha/1 -> MATLAB Function/1(u)

== system Open_loop_BPS_comparsion2/linear BPS ==
  note: X_dot
  note: X
  note: U
  note: U
  note: X_dot
  note: X
  Alpha : Inport
  Beta : Inport  Port=2
  Integrator : Integrator
  Integrator1 : Integrator
  MATLAB Function : MATLAB Function  TreatAsAtomicUnit=on
  MATLAB Function1 : MATLAB Function  TreatAsAtomicUnit=on
  MATLAB Function2 : MATLAB Function  TreatAsAtomicUnit=on
  MATLAB Function3 : MATLAB Function  TreatAsAtomicUnit=on
  MATLAB Function4 : MATLAB Function  TreatAsAtomicUnit=on
  MATLAB Function5 : MATLAB Function  TreatAsAtomicUnit=on
  Sum : Sum  Inputs=|++
  Sum1 : Sum  Inputs=|++
  X : Outport
  Y : Outport  Port=2
  wires:
  MATLAB Function2/1(y) -> Sum/1
  MATLAB Function/1(y) -> Sum/2
  MATLAB Function1/1(y) -> X/1
  Sum1/1 -> Integrator1/1
  Integrator/1 -> MATLAB Function2/1(x), MATLAB Function1/1(x)
  Sum/1 -> Integrator/1
  MATLAB Function5/1(y) -> Sum1/2
  MATLAB Function4/1(y) -> Y/1
  Beta/1 -> MATLAB Function3/1(u)
  Integrator1/1 -> MATLAB Function5/1(x), MATLAB Function4/1(x)
  MATLAB Function3/1(y) -> Sum1/1
  Alpha/1 -> MATLAB Function/1(u)
